simulink model "dcom7"  (Simulink 7.8)
settings: Solver=ode45  StartTime=0.0  StopTime=10  RelTol=1e-3
libraries: commblkcod2 x2, commchan3 x2, commsink2 x2, commrandsrc2 x1
settings Model: Creator=DJSCE.Student  LastModifiedBy=DJSCE.Student

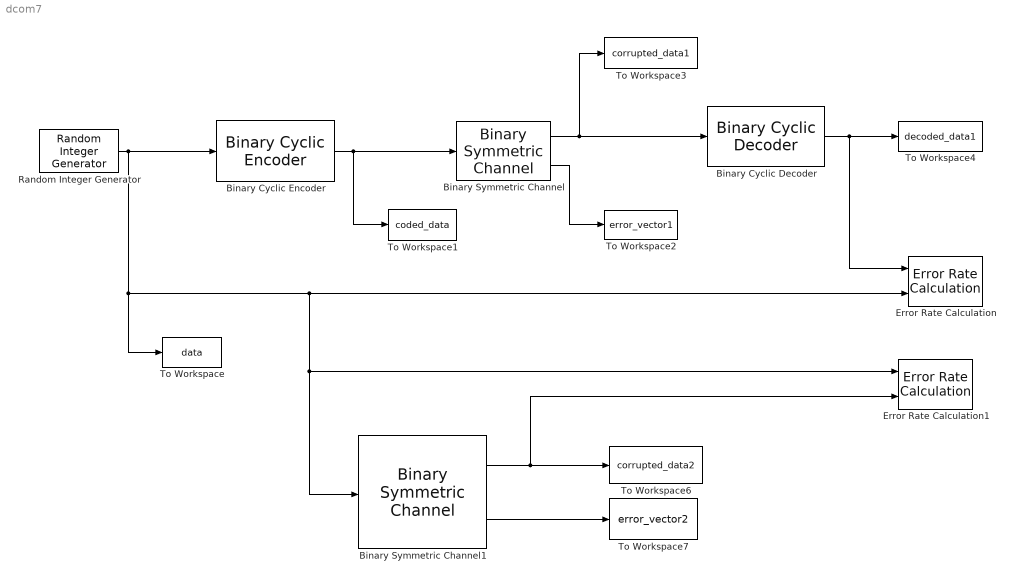
== system dcom7 ==
  Binary Cyclic Decoder : commblkcod2/Binary Cyclic Decoder  n=7  p=4
  Binary Cyclic Encoder : commblkcod2/Binary Cyclic Encoder  n=7  p=4
  Binary Symmetric Channel : commchan3/Binary Symmetric Channel  P=0.6  s=71  E=on  outDtype=double
  Binary Symmetric Channel1 : commchan3/Binary Symmetric Channel  P=0.6  s=71  E=on  outDtype=double
  Error Rate Calculation : commsink2/Error Rate Calculation  N=0  st_delay=0  cp_mode=Entire frame  subframe=[]  PMode=Workspace  WsName=ErrorVec  RsMode2=off  stop=off  numErr=100  maxBits=1e6
  Error Rate Calculation1 : commsink2/Error Rate Calculation  N=0  st_delay=0  cp_mode=Entire frame  subframe=[]  PMode=Workspace  WsName=ErrorVec1  RsMode2=off  stop=off  numErr=100  maxBits=1e6
  Random Integer Generator : commrandsrc2/Random Integer Generator  mul=2  seed=0  Ts=1  frameBased=on  sampPerFrame=4  orient=off  outDataType=double
  To Workspace : ToWorkspace  VariableName=data  SampleTime=-1  SaveFormat=Structure
  To Workspace1 : ToWorkspace  VariableName=coded_data  SampleTime=-1  SaveFormat=Structure
  To Workspace2 : ToWorkspace  VariableName=error_vector1  SampleTime=-1  SaveFormat=Structure
  To Workspace3 : ToWorkspace  VariableName=corrupted_data1  SampleTime=-1  SaveFormat=Structure
  To Workspace4 : ToWorkspace  VariableName=decoded_data1  SampleTime=-1  SaveFormat=Structure
  To Workspace6 : ToWorkspace  VariableName=corrupted_data2  SampleTime=-1  SaveFormat=Structure
  To Workspace7 : ToWorkspace  VariableName=error_vector2  SampleTime=-1  SaveFormat=Structure
  wires:
  Random Integer Generator/1 -> Binary Cyclic Encoder/1, To Workspace/1, Error Rate Calculation/2, Binary Symmetric Channel1/1, Error Rate Calculation1/1
  Binary Cyclic Encoder/1 -> Binary Symmetric Channel/1, To Workspace1/1
  Binary Symmetric Channel/1 -> Binary Cyclic Decoder/1, To Workspace3/1
  Binary Symmetric Channel/2 -> To Workspace2/1
  Binary Cyclic Decoder/1 -> To Workspace4/1, Error Rate Calculation/1
  Binary Symmetric Channel1/2 -> To Workspace7/1
  Binary Symmetric Channel1/1 -> To Workspace6/1, Error Rate Calculation1/2
